simulink model "Plant_controller_1"  (R2017a)
settings: Solver=VariableStepAuto  StartTime=0.0  StopTime=500  RelTol=1e-3
libraries: simulink_extras x1
settings Model: Creator=Jaydeep  LastModifiedBy=Jaydeep

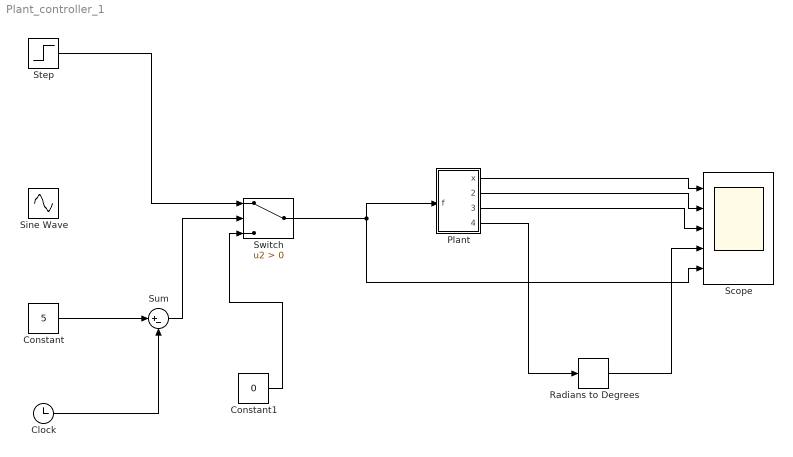
== system Plant_controller_1 ==
  Clock : Clock
  Constant : Constant  Value=5
  Constant1 : Constant  Value=0
  Plant : Subsystem
  Radians to Degrees : simulink_extras/Transformations/Radians to Degrees
  Scope : Scope  NumInputPorts=5
  Sine Wave : Sin  Frequency=50  SampleTime=0
  Step : Step  SampleTime=0
  Sum : Sum  Inputs=|+-
  Switch : Switch  Criteria=u2 > Threshold
  wires:
  Plant/1(x) -> Scope/1
  Plant/2(xdot) -> Scope/2
  Plant/3("tdot ") -> Scope/3
  Clock/1 -> Sum/2
  Constant/1 -> Sum/1
  Sum/1 -> Switch/2
  Constant1/1 -> Switch/3
  Switch/1 -> Plant/1(f), Scope/5
  Step/1 -> Switch/1
  Plant/4("theta ") -> Radians to Degrees/1
  Radians to Degrees/1 -> Scope/4

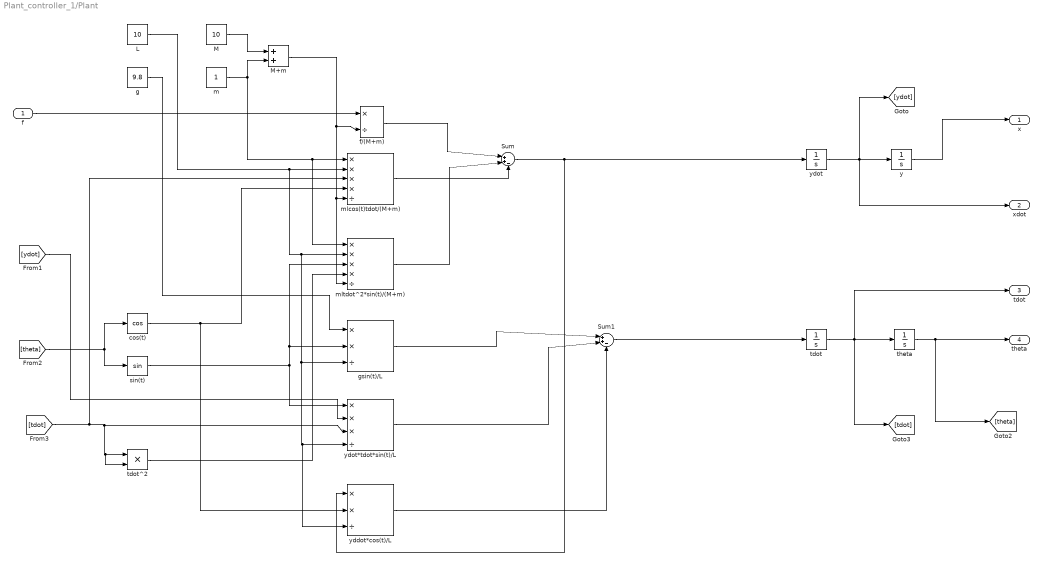
== system Plant_controller_1/Plant ==
  f : Inport
  L : Constant  Value=10
  M : Constant  Value=10
  "M+m " : Sum
  Sum : Sum  Inputs=|++-
  Sum1 : Sum  Inputs=|++-
  cos(t) : Trigonometry  Operator=cos
  f/(M+m) : Product  Inputs=*/
  g : Constant  Value=9.8
  gsin(t)/L : Product  Inputs=**/
  "m " : Constant
  mlcos(t)tdot/(M+m) : Product  Inputs=****/
  mltdot^2*sin(t)/(M+m) : Product  Inputs=****/
  "sin(t) " : Trigonometry
  tdot : Integrator
  tdot^2 : Product
  theta : Integrator  InitialCondition=pi  UpperSaturationLimit=30  LowerSaturationLimit=-30
  y : Integrator
  yddot*cos(t)/L : Product  Inputs=**/
  "ydot " : Integrator
  ydot*tdot*sin(t)/L : Product  Inputs=***/
  x : Outport
  xdot : Outport  Port=2
  "tdot " : Outport  Port=3
  "theta " : Outport  Port=4
  wires:
  tdot^2/1 -> mltdot^2*sin(t)/(M+m)/4
  "ydot "/1 -> xdot/1, [ydot], y/1
  Sum/1 -> yddot*cos(t)/L/1, "ydot "/1
  mlcos(t)tdot/(M+m)/1 -> Sum/3
  theta/1 -> "theta "/1, [theta]
  f/(M+m)/1 -> Sum/1
  g/1 -> gsin(t)/L/1
  "sin(t) "/1 -> ydot*tdot*sin(t)/L/1, gsin(t)/L/2, mltdot^2*sin(t)/(M+m)/3
  tdot/1 -> "tdot "/1, [tdot], theta/1
  L/1 -> yddot*cos(t)/L/3, ydot*tdot*sin(t)/L/4, gsin(t)/L/3, mltdot^2*sin(t)/(M+m)/2, mlcos(t)tdot/(M+m)/2
  gsin(t)/L/1 -> Sum1/1
  cos(t)/1 -> yddot*cos(t)/L/2, mlcos(t)tdot/(M+m)/4
  f/1 -> f/(M+m)/1
  mltdot^2*sin(t)/(M+m)/1 -> Sum/2
  [tdot] -> ydot*tdot*sin(t)/L/3, tdot^2/2, tdot^2/1, mlcos(t)tdot/(M+m)/3
  M/1 -> "M+m "/1
  [theta] -> cos(t)/1, "sin(t) "/1
  Sum1/1 -> tdot/1
  "m "/1 -> mltdot^2*sin(t)/(M+m)/1, mlcos(t)tdot/(M+m)/1, "M+m "/2
  "M+m "/1 -> mltdot^2*sin(t)/(M+m)/5, mlcos(t)tdot/(M+m)/5, f/(M+m)/2
  ydot*tdot*sin(t)/L/1 -> Sum1/2
  yddot*cos(t)/L/1 -> Sum1/3
  y/1 -> x/1
  [ydot] -> ydot*tdot*sin(t)/L/2
